simulink model "taghriban_kamel_faghat_bare3yekam_Ero"  (Simulink 7.3)
settings: Solver=ode45  StartTime=0.0  StopTime=.6  RelTol=1e-3
undefined symbols (not defined in the file or in its folder): x
libraries: powerlib x218, powerlib_extras x125
(part 1 of 2)
settings Model: Creator=me  LastModifiedBy=me

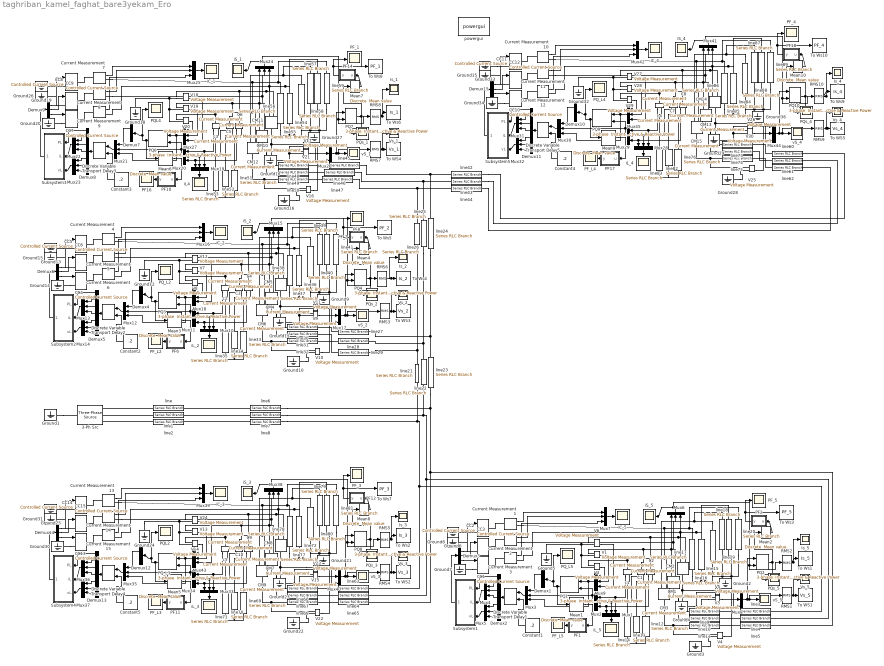
== system taghriban_kamel_faghat_bare3yekam_Ero ==
  3-Ph Src : powerlib/Electrical Sources/Three-Phase Source  DialogController=POWERSYS.PowerSysDialog  SystemSampleTime=-1  Voltage=380  PhaseAngle=0  Frequency=50  InternalConnection=Yn  SpecifyImpedance=on  Resistance=0.8929  Inductance=16.58e-3  ShortCircuitLevel=100e6  BaseVoltage=380  XRratio=7
  C{1..10} (10 alike) : powerlib/Measurements/Current Measurement  DialogController=POWERSYS.PowerSysDialog  SystemSampleTime=-1  PhasorSimulation=off  OutputType=Complex  PSBequivalent=0
  CC{1..15} (15 alike) : powerlib/Electrical Sources/Controlled Current Source  DialogController=POWERSYS.PowerSysDialog  SystemSampleTime=-1  Initialize=on  Source_Type=AC  Amplitude=0  Phase=0  Frequency=0  Measurements=None
  CM{1..15} (15 alike) : powerlib/Measurements/Current Measurement  DialogController=POWERSYS.PowerSysDialog  SystemSampleTime=-1  PhasorSimulation=off  OutputType=Complex  PSBequivalent=0
  Constant{1..5} (5 alike) : Constant  Value=.2  OutDataType=sfix(16)  OutScaling=2^0
  Current Measurement{1..15} (15 alike) : powerlib/Measurements/Current Measurement  DialogController=POWERSYS.PowerSysDialog  SystemSampleTime=-1  PhasorSimulation=off  OutputType=Complex  PSBequivalent=0
  Demux{1,4,7,10,12} (5 alike) : Demux  Outputs=2
  Demux{2,5,8,11,13} (5 alike) : Demux  Outputs=7
  Demux{3,6,9,14..15} (5 alike) : Demux  Outputs=3
  Discrete Variable Transport Delay{1..5} (5 alike) : powerlib_extras/Discrete  Control Blocks/Discrete Variable Transport Delay  DialogController=POWERSYS.PowerSysDialog  SystemSampleTime=-1  MaxDelay=1/40  InitialValue=0  Ts=50e-6
  Ground{1..36} (36 alike) : powerlib/Elements/Ground  DialogController=POWERSYS.PowerSysDialog  PhysicalDomain=powersysdomain  SubClassName=unknown  LeftPortType=p1  RightPortType=p1  LConnTagsString=a
  Is_{1..5} (5 alike) : Scope
      Is_1 settings: TimeRange=0.25  YMin=-1  YMax=1  SaveName=ScopeData21
      Is_2 settings: TimeRange=0.25  YMin=-1  YMax=1  SaveName=ScopeData11
      Is_3 settings: TimeRange=0.25  YMin=-1  YMax=1  SaveName=ScopeData50
      Is_4 settings: TimeRange=0.25  YMin=-1  YMax=1  SaveName=ScopeData44
      Is_5 settings: TimeRange=0.25  YMin=-1  YMax=1
  Mean{1..10} (10 alike) : powerlib_extras/Discrete Measurements/Discrete  Mean value  DialogController=POWERSYS.PowerSysDialog  SystemSampleTime=-1  Freq=60  Vinit=0  Ts=50e-6
  Mux{1..45} (45 alike) : Mux  Inputs=3
  PF1 : Stateflow chart
  PF10 : Stateflow chart
  PF11 : Stateflow chart
  PF12 : Stateflow chart
  PF14 : Stateflow chart
  PF16 : Scope
      settings: YMin=0.9675  YMax=0.9975  SaveName=ScopeData28
  PF17 : Stateflow chart
  PF18 : Stateflow chart
  PF2 : Stateflow chart
  PF6 : Stateflow chart
  PF8 : Scope
      settings: YMin=0.9961  YMax=0.9978  SaveName=ScopeData12
  PF_{1,3..5} (4 alike) : Scope
      PF_1 settings: YMin=0.957  YMax=0.965  SaveName=ScopeData22
      PF_3 settings: YMin=0.9961  YMax=0.9978  SaveName=ScopeData23
      PF_4 settings: YMin=0.9961  YMax=0.9978  SaveName=ScopeData45
      PF_5 settings: YMin=0.9961  YMax=0.9978  SaveName=ScopeData2
  PF_2 : Stateflow chart
  PF_L{2..5} (4 alike) : Scope
      PF_L2 settings: YMin=0.9675  YMax=0.9975  SaveName=ScopeData13
      PF_L3 settings: YMin=0.9675  YMax=0.9975  SaveName=ScopeData24
      PF_L4 settings: YMin=0.9675  YMax=0.9975  SaveName=ScopeData46
      PF_L5 settings: YMin=0.9675  YMax=0.9975  SaveName=ScopeData3
  PQ{1..4,6..10} (9 alike) : powerlib_extras/Measurements/3-phase  Instantaneous  Active & Reactive Power  DialogController=POWERSYS.PowerSysDialog  SystemSampleTime=-1
  PQL2 : Scope
      settings: TimeRange=0.2  YMin=-2e+008  YMax=9e+008  SaveName=ScopeData25
  PQL4 : Scope
      settings: TimeRange=0.2  YMin=-2e+008  YMax=9e+008  SaveName=ScopeData29
  PQ_L2 : Scope
      settings: TimeRange=0.2  YMin=-2e+008  YMax=9e+008  SaveName=ScopeData14
  PQ_L3 : powerlib_extras/Measurements/3-phase  Instantaneous  Active & Reactive Power  DialogController=POWERSYS.PowerSysDialog  SystemSampleTime=-1
  PQ_L4 : Scope
      settings: TimeRange=0.2  YMin=-2e+008  YMax=9e+008  SaveName=ScopeData47
  PQ_L5 : Scope
      settings: TimeRange=0.2  YMin=-2e+008  YMax=9e+008  SaveName=ScopeData4
  PQs_{1..5} (5 alike) : Scope
      PQs_1 settings: TimeRange=0.25  YMin=-250  YMax=4000  SaveName=ScopeData30
      PQs_2 settings: TimeRange=0.25  YMin=-250  YMax=4000  SaveName=ScopeData15
      PQs_3 settings: TimeRange=0.25  YMin=-250  YMax=4000  SaveName=ScopeData26
      PQs_4 settings: TimeRange=0.25  YMin=-250  YMax=4000  SaveName=ScopeData48
      PQs_5 settings: TimeRange=0.25  YMin=-250  YMax=4000  SaveName=ScopeData5
  RMS{1..10} (10 alike) : powerlib_extras/Measurements/RMS  DialogController=POWERSYS.PowerSysDialog  SystemSampleTime=-1  f1=50
  Subsystem1 : Subsystem
  Subsystem2 : Subsystem
  Subsystem3 : Subsystem
  Subsystem4 : Subsystem
  Subsystem5 : Subsystem
  To WS1 : ToWorkspace  VariableName=Vs_5  SampleTime=.01  SaveFormat=Array
  To WS2 : ToWorkspace  VariableName=Vs_3  SampleTime=.01  SaveFormat=Array
  To WS3 : ToWorkspace  VariableName=Vs_2  SampleTime=.01  SaveFormat=Array
  To WS4 : ToWorkspace  VariableName=Vs_1  SampleTime=.01  SaveFormat=Array
  To WS5 : ToWorkspace  VariableName=Vs_4  SampleTime=.01  SaveFormat=Array
  To Ws1 : ToWorkspace  VariableName=Is_5  SampleTime=.01  SaveFormat=Array
  To Ws10 : ToWorkspace  VariableName=PF_4  SampleTime=.01  SaveFormat=Array
  To Ws2 : ToWorkspace  VariableName=Is_3  SampleTime=.01  SaveFormat=Array
  To Ws3 : ToWorkspace  VariableName=PF_5  SampleTime=.01  SaveFormat=Array
  To Ws4 : ToWorkspace  VariableName=Is_2  SampleTime=.01  SaveFormat=Array
  To Ws5 : ToWorkspace  VariableName=PF_2  SampleTime=.01  SaveFormat=Array
  To Ws6 : ToWorkspace  VariableName=Is_1  SampleTime=.01  SaveFormat=Array
  To Ws7 : ToWorkspace  VariableName=PF_3  SampleTime=.01  SaveFormat=Array
  To Ws8 : ToWorkspace  VariableName=PF_1  SampleTime=.01  SaveFormat=Array
  To Ws9 : ToWorkspace  VariableName=Is_4  SampleTime=.01  SaveFormat=Array
  V{1..30} (30 alike) : powerlib/Measurements/Voltage Measurement  DialogController=POWERSYS.PowerSysDialog  SystemSampleTime=-1  PhasorSimulation=off  OutputType=Complex  PSBequivalent=0
  Vs_{1..5} (5 alike) : Scope
      Vs_1 settings: TimeRange=0.25  YMin=217.8  YMax=217.93  SaveName=ScopeData36
      Vs_2 settings: TimeRange=0.25  YMin=217.8  YMax=217.93  SaveName=ScopeData16
      Vs_3 settings: TimeRange=0.25  YMin=217.8  YMax=217.93  SaveName=ScopeData51
      Vs_4 settings: TimeRange=0.25  YMin=217.8  YMax=217.93  SaveName=ScopeData49
      Vs_5 settings: TimeRange=0.25  YMin=217.8  YMax=217.93  SaveName=ScopeData6
  c{1..5} (5 alike) : powerlib/Measurements/Current Measurement  DialogController=POWERSYS.PowerSysDialog  SystemSampleTime=-1  PhasorSimulation=off  OutputType=Complex  PSBequivalent=0
  iC_{1..5} (5 alike) : Scope
      iC_1 settings: TimeRange=0.15  YMin=-10  YMax=10  SaveName=ScopeData38
      iC_2 settings: TimeRange=0.15  YMin=-10  YMax=10  SaveName=ScopeData17
      iC_3 settings: TimeRange=0.15  YMin=-10  YMax=10  SaveName=ScopeData27
      iC_4 settings: TimeRange=0.15  YMin=-10  YMax=10  SaveName=ScopeData52
      iC_5 settings: TimeRange=0.15  YMin=-10  YMax=10  SaveName=ScopeData7
  iL4 : Scope
      settings: TimeRange=0.15  YMin=-4000  YMax=3500  SaveName=ScopeData39
  iL_{2..5} (4 alike) : Scope
      iL_2 settings: TimeRange=0.15  YMin=-4000  YMax=3500  SaveName=ScopeData18
      iL_3 settings: TimeRange=0.15  YMin=-4000  YMax=3500  SaveName=ScopeData37
      iL_4 settings: TimeRange=0.15  YMin=-4000  YMax=3500  SaveName=ScopeData53
      iL_5 settings: TimeRange=0.15  YMin=-4000  YMax=3500  SaveName=ScopeData8
  iS_{1..5} (5 alike) : Scope
      iS_1 settings: TimeRange=0.2  YMin=-15  YMax=15  SaveName=ScopeData42
      iS_2 settings: TimeRange=0.2  YMin=-17.5  YMax=17.5  SaveName=ScopeData19
      iS_3 settings: TimeRange=0.25  YMin=-15  YMax=15  SaveName=ScopeData40
      iS_4 settings: TimeRange=0.45  YMin=-10  YMax=10  SaveName=ScopeData54
      iS_5 settings: TimeRange=0.45  YMin=-12.5  YMax=12.5  SaveName=ScopeData9
  line : powerlib/Elements/Series RLC Branch  DialogController=POWERSYS.PowerSysDialog  PhysicalDomain=powersysdomain  SubClassName=unknown  LeftPortType=p1  RightPortType=p1  LConnTagsString=__new0  RConnTagsString=__new0  BranchType=RL  Resistance=.08  Inductance=.06/(100*pi)  SetiL0=off  InitialCurrent=0  Capacitance=1.0  Setx0=off  InitialVoltage=0  Measurements=None
  line1 : powerlib/Elements/Series RLC Branch  DialogController=POWERSYS.PowerSysDialog  PhysicalDomain=powersysdomain  SubClassName=unknown  LeftPortType=p1  RightPortType=p1  LConnTagsString=__new0  RConnTagsString=__new0  BranchType=RL  Resistance=.08  Inductance=.06/(100*pi)  SetiL0=off  InitialCurrent=0  Capacitance=1.0  Setx0=off  InitialVoltage=0  Measurements=None
  line{9..11,30..32,48..50,66..68,73..75} (15 alike) : powerlib/Elements/Series RLC Branch  DialogController=POWERSYS.PowerSysDialog  PhysicalDomain=powersysdomain  SubClassName=unknown  LeftPortType=p1  RightPortType=p1  LConnTagsString=__new0  RConnTagsString=__new0  BranchType=RL  Resistance=.1  Inductance=.08/(100*pi)  SetiL0=off  InitialCurrent=0  Capacitance=1.0  Setx0=off  InitialVoltage=0  Measurements=None
  line12 : powerlib/Elements/Series RLC Branch  DialogController=POWERSYS.PowerSysDialog  PhysicalDomain=powersysdomain  SubClassName=unknown  LeftPortType=p1  RightPortType=p1  LConnTagsString=__new0  RConnTagsString=__new0  BranchType=RL  Resistance=24  Inductance=19/(100*pi)  SetiL0=off  InitialCurrent=0  Capacitance=1.0  Setx0=off  InitialVoltage=0  Measurements=None
  line13 : powerlib/Elements/Series RLC Branch  DialogController=POWERSYS.PowerSysDialog  PhysicalDomain=powersysdomain  SubClassName=unknown  LeftPortType=p1  RightPortType=p1  LConnTagsString=__new0  RConnTagsString=__new0  BranchType=Open circuit  Resistance=50  Inductance=50/(100*pi)  SetiL0=off  InitialCurrent=0  Capacitance=1/(100*pi)  Setx0=off  InitialVoltage=0  Measurements=None
  line14 : powerlib/Elements/Series RLC Branch  DialogController=POWERSYS.PowerSysDialog  PhysicalDomain=powersysdomain  SubClassName=unknown  LeftPortType=p1  RightPortType=p1  LConnTagsString=__new0  RConnTagsString=__new0  BranchType=RL  Resistance=10  Inductance=30/(100*pi)  SetiL0=off  InitialCurrent=0  Capacitance=1/(100*pi)  Setx0=off  InitialVoltage=0  Measurements=None
  line{15..17,36..38,54..56,72,77..78,84..86} (15 alike) : powerlib/Elements/Series RLC Branch  DialogController=POWERSYS.PowerSysDialog  PhysicalDomain=powersysdomain  SubClassName=unknown  LeftPortType=p1  RightPortType=p1  LConnTagsString=__new0  RConnTagsString=__new0  BranchType=R  Resistance=100  Inductance=.04/(100*pi)  SetiL0=off  InitialCurrent=0  Capacitance=1.0  Setx0=off  InitialVoltage=0  Measurements=None
  line{18..20,39..41,57..59,79..81,87..89} (15 alike) : powerlib/Elements/Series RLC Branch  DialogController=POWERSYS.PowerSysDialog  PhysicalDomain=powersysdomain  SubClassName=unknown  LeftPortType=p1  RightPortType=p1  LConnTagsString=__new0  RConnTagsString=__new0  BranchType=C  Resistance=100  Inductance=.04/(100*pi)  SetiL0=off  InitialCurrent=0  Capacitance=1/(10000*pi)  Setx0=off  InitialVoltage=0  Measurements=None
  line2 : powerlib/Elements/Series RLC Branch  DialogController=POWERSYS.PowerSysDialog  PhysicalDomain=powersysdomain  SubClassName=unknown  LeftPortType=p1  RightPortType=p1  LConnTagsString=__new0  RConnTagsString=__new0  BranchType=RL  Resistance=.08  Inductance=.06/(100*pi)  SetiL0=off  InitialCurrent=0  Capacitance=1.0  Setx0=off  InitialVoltage=0  Measurements=None
  line21 : powerlib/Elements/Series RLC Branch  DialogController=POWERSYS.PowerSysDialog  PhysicalDomain=powersysdomain  SubClassName=unknown  LeftPortType=p1  RightPortType=p1  LConnTagsString=__new0  RConnTagsString=__new0  BranchType=RL  Resistance=.11  Inductance=.08/(100*pi)  SetiL0=off  InitialCurrent=0  Capacitance=1.0  Setx0=off  InitialVoltage=0  Measurements=None
  line22 : powerlib/Elements/Series RLC Branch  DialogController=POWERSYS.PowerSysDialog  PhysicalDomain=powersysdomain  SubClassName=unknown  LeftPortType=p1  RightPortType=p1  LConnTagsString=__new0  RConnTagsString=__new0  BranchType=RL  Resistance=.11  Inductance=.08/(100*pi)  SetiL0=off  InitialCurrent=0  Capacitance=1.0  Setx0=off  InitialVoltage=0  Measurements=None
  line23 : powerlib/Elements/Series RLC Branch  DialogController=POWERSYS.PowerSysDialog  PhysicalDomain=powersysdomain  SubClassName=unknown  LeftPortType=p1  RightPortType=p1  LConnTagsString=__new0  RConnTagsString=__new0  BranchType=RL  Resistance=.11  Inductance=.08/(100*pi)  SetiL0=off  InitialCurrent=0  Capacitance=1.0  Setx0=off  InitialVoltage=0  Measurements=None
  line24 : powerlib/Elements/Series RLC Branch  DialogController=POWERSYS.PowerSysDialog  PhysicalDomain=powersysdomain  SubClassName=unknown  LeftPortType=p1  RightPortType=p1  LConnTagsString=__new0  RConnTagsString=__new0  BranchType=RL  Resistance=.06  Inductance=.04/(100*pi)  SetiL0=off  InitialCurrent=0  Capacitance=1.0  Setx0=off  InitialVoltage=0  Measurements=None
  line25 : powerlib/Elements/Series RLC Branch  DialogController=POWERSYS.PowerSysDialog  PhysicalDomain=powersysdomain  SubClassName=unknown  LeftPortType=p1  RightPortType=p1  LConnTagsString=__new0  RConnTagsString=__new0  BranchType=RL  Resistance=.06  Inductance=.04/(100*pi)  SetiL0=off  InitialCurrent=0  Capacitance=1.0  Setx0=off  InitialVoltage=0  Measurements=None
  line26 : powerlib/Elements/Series RLC Branch  DialogController=POWERSYS.PowerSysDialog  PhysicalDomain=powersysdomain  SubClassName=unknown  LeftPortType=p1  RightPortType=p1  LConnTagsString=__new0  RConnTagsString=__new0  BranchType=RL  Resistance=.06  Inductance=.04/(100*pi)  SetiL0=off  InitialCurrent=0  Capacitance=1.0  Setx0=off  InitialVoltage=0  Measurements=None
  line{3,27,45,60,63} (5 alike) : powerlib/Elements/Series RLC Branch  DialogController=POWERSYS.PowerSysDialog  PhysicalDomain=powersysdomain  SubClassName=unknown  LeftPortType=p1  RightPortType=p1  LConnTagsString=__new0  RConnTagsString=__new0  BranchType=R  Resistance=.000000000001  Inductance=1.0  SetiL0=off  InitialCurrent=0  Capacitance=1.0  Setx0=off  InitialVoltage=0  Measurements=None
  line{4,28,46,61,64} (5 alike) : powerlib/Elements/Series RLC Branch  DialogController=POWERSYS.PowerSysDialog  PhysicalDomain=powersysdomain  SubClassName=unknown  LeftPortType=p1  RightPortType=p1  LConnTagsString=__new0  RConnTagsString=__new0  BranchType=R  Resistance=.0000000001  Inductance=1.0  SetiL0=off  InitialCurrent=0  Capacitance=1.0  Setx0=off  InitialVoltage=0  Measurements=None
  line{5,29,47,62,65} (5 alike) : powerlib/Elements/Series RLC Branch  DialogController=POWERSYS.PowerSysDialog  PhysicalDomain=powersysdomain  SubClassName=unknown  LeftPortType=p1  RightPortType=p1  LConnTagsString=__new0  RConnTagsString=__new0  BranchType=R  Resistance=.0000000000001  Inductance=1.0  SetiL0=off  InitialCurrent=0  Capacitance=1.0  Setx0=off  InitialVoltage=0  Measurements=None
  line33 : powerlib/Elements/Series RLC Branch  DialogController=POWERSYS.PowerSysDialog  PhysicalDomain=powersysdomain  SubClassName=unknown  LeftPortType=p1  RightPortType=p1  LConnTagsString=__new0  RConnTagsString=__new0  BranchType=RL  Resistance=14  Inductance=29/(100*pi)  SetiL0=off  InitialCurrent=0  Capacitance=1.0  Setx0=off  InitialVoltage=0  Measurements=None
  line34 : powerlib/Elements/Series RLC Branch  DialogController=POWERSYS.PowerSysDialog  PhysicalDomain=powersysdomain  SubClassName=unknown  LeftPortType=p1  RightPortType=p1  LConnTagsString=__new0  RConnTagsString=__new0  BranchType=RC  Resistance=23  Inductance=50/(100*pi)  SetiL0=off  InitialCurrent=0  Capacitance=1/(1200*pi)  Setx0=off  InitialVoltage=0  Measurements=None
  line35 : powerlib/Elements/Series RLC Branch  DialogController=POWERSYS.PowerSysDialog  PhysicalDomain=powersysdomain  SubClassName=unknown  LeftPortType=p1  RightPortType=p1  LConnTagsString=__new0  RConnTagsString=__new0  BranchType=Open circuit  Resistance=10  Inductance=30/(100*pi)  SetiL0=off  InitialCurrent=0  Capacitance=1/(100*pi)  Setx0=off  InitialVoltage=0  Measurements=None
  line42 : powerlib/Elements/Series RLC Branch  DialogController=POWERSYS.PowerSysDialog  PhysicalDomain=powersysdomain  SubClassName=unknown  LeftPortType=p1  RightPortType=p1  LConnTagsString=__new0  RConnTagsString=__new0  BranchType=RL  Resistance=.05  Inductance=.04/(100*pi)  SetiL0=off  InitialCurrent=0  Capacitance=1.0  Setx0=off  InitialVoltage=0  Measurements=None
  line43 : powerlib/Elements/Series RLC Branch  DialogController=POWERSYS.PowerSysDialog  PhysicalDomain=powersysdomain  SubClassName=unknown  LeftPortType=p1  RightPortType=p1  LConnTagsString=__new0  RConnTagsString=__new0  BranchType=RL  Resistance=.05  Inductance=.04/(100*pi)  SetiL0=off  InitialCurrent=0  Capacitance=1.0  Setx0=off  InitialVoltage=0  Measurements=None
  line44 : powerlib/Elements/Series RLC Branch  DialogController=POWERSYS.PowerSysDialog  PhysicalDomain=powersysdomain  SubClassName=unknown  LeftPortType=p1  RightPortType=p1  LConnTagsString=__new0  RConnTagsString=__new0  BranchType=RL  Resistance=.05  Inductance=.04/(100*pi)  SetiL0=off  InitialCurrent=0  Capacitance=1.0  Setx0=off  InitialVoltage=0  Measurements=None
  line51 : powerlib/Elements/Series RLC Branch  DialogController=POWERSYS.PowerSysDialog  PhysicalDomain=powersysdomain  SubClassName=unknown  LeftPortType=p1  RightPortType=p1  LConnTagsString=__new0  RConnTagsString=__new0  BranchType=RLC  Resistance=24  Inductance=39/(100*pi)  SetiL0=off  InitialCurrent=0  Capacitance=1/(1200*pi)  Setx0=off  InitialVoltage=0  Measurements=None
  line52 : powerlib/Elements/Series RLC Branch  DialogController=POWERSYS.PowerSysDialog  PhysicalDomain=powersysdomain  SubClassName=unknown  LeftPortType=p1  RightPortType=p1  LConnTagsString=__new0  RConnTagsString=__new0  BranchType=RC  Resistance=50  Inductance=50/(100*pi)  SetiL0=off  InitialCurrent=0  Capacitance=1/(1000*pi)  Setx0=off  InitialVoltage=0  Measurements=None
  line53 : powerlib/Elements/Series RLC Branch  DialogController=POWERSYS.PowerSysDialog  PhysicalDomain=powersysdomain  SubClassName=unknown  LeftPortType=p1  RightPortType=p1  LConnTagsString=__new0  RConnTagsString=__new0  BranchType=RL  Resistance=5  Inductance=30/(100*pi)  SetiL0=off  InitialCurrent=0  Capacitance=1/(100*pi)  Setx0=off  InitialVoltage=0  Measurements=None
  line6 : powerlib/Elements/Series RLC Branch  DialogController=POWERSYS.PowerSysDialog  PhysicalDomain=powersysdomain  SubClassName=unknown  LeftPortType=p1  RightPortType=p1  LConnTagsString=__new0  RConnTagsString=__new0  BranchType=RL  Resistance=.03  Inductance=.02/(100*pi)  SetiL0=off  InitialCurrent=0  Capacitance=1.0  Setx0=off  InitialVoltage=0  Measurements=None
  line69 : powerlib/Elements/Series RLC Branch  DialogController=POWERSYS.PowerSysDialog  PhysicalDomain=powersysdomain  SubClassName=unknown  LeftPortType=p1  RightPortType=p1  LConnTagsString=__new0  RConnTagsString=__new0  BranchType=RL  Resistance=24  Inductance=9/(100*pi)  SetiL0=off  InitialCurrent=0  Capacitance=1.0  Setx0=off  InitialVoltage=0  Measurements=None
  line7 : powerlib/Elements/Series RLC Branch  DialogController=POWERSYS.PowerSysDialog  PhysicalDomain=powersysdomain  SubClassName=unknown  LeftPortType=p1  RightPortType=p1  LConnTagsString=__new0  RConnTagsString=__new0  BranchType=RL  Resistance=.03  Inductance=.02/(100*pi)  SetiL0=off  InitialCurrent=0  Capacitance=1.0  Setx0=off  InitialVoltage=0  Measurements=None
  line70 : powerlib/Elements/Series RLC Branch  DialogController=POWERSYS.PowerSysDialog  PhysicalDomain=powersysdomain  SubClassName=unknown  LeftPortType=p1  RightPortType=p1  LConnTagsString=__new0  RConnTagsString=__new0  BranchType=RLC  Resistance=15  Inductance=50/(100*pi)  SetiL0=off  InitialCurrent=0  Capacitance=26/(100*pi)  Setx0=off  InitialVoltage=0  Measurements=None
  line71 : powerlib/Elements/Series RLC Branch  DialogController=POWERSYS.PowerSysDialog  PhysicalDomain=powersysdomain  SubClassName=unknown  LeftPortType=p1  RightPortType=p1  LConnTagsString=__new0  RConnTagsString=__new0  BranchType=L  Resistance=10  Inductance=30/(100*pi)  SetiL0=off  InitialCurrent=0  Capacitance=1/(100*pi)  Setx0=off  InitialVoltage=0  Measurements=None
  line76 : powerlib/Elements/Series RLC Branch  DialogController=POWERSYS.PowerSysDialog  PhysicalDomain=powersysdomain  SubClassName=unknown  LeftPortType=p1  RightPortType=p1  LConnTagsString=__new0  RConnTagsString=__new0  BranchType=RL  Resistance=24  Inductance=41/(100*pi)  SetiL0=off  InitialCurrent=0  Capacitance=1.0  Setx0=off  InitialVoltage=0  Measurements=None
  line8 : powerlib/Elements/Series RLC Branch  DialogController=POWERSYS.PowerSysDialog  PhysicalDomain=powersysdomain  SubClassName=unknown  LeftPortType=p1  RightPortType=p1  LConnTagsString=__new0  RConnTagsString=__new0  BranchType=RL  Resistance=.03  Inductance=.02/(100*pi)  SetiL0=off  InitialCurrent=0  Capacitance=1.0  Setx0=off  InitialVoltage=0  Measurements=None
  line82 : powerlib/Elements/Series RLC Branch  DialogController=POWERSYS.PowerSysDialog  PhysicalDomain=powersysdomain  SubClassName=unknown  LeftPortType=p1  RightPortType=p1  LConnTagsString=__new0  RConnTagsString=__new0  BranchType=RLC  Resistance=7  Inductance=50/(100*pi)  SetiL0=off  InitialCurrent=0  Capacitance=1/(1000*pi)  Setx0=off  InitialVoltage=0  Measurements=None
  line83 : powerlib/Elements/Series RLC Branch  DialogController=POWERSYS.PowerSysDialog  PhysicalDomain=powersysdomain  SubClassName=unknown  LeftPortType=p1  RightPortType=p1  LConnTagsString=__new0  RConnTagsString=__new0  BranchType=RL  Resistance=10  Inductance=20/(100*pi)  SetiL0=off  InitialCurrent=0  Capacitance=1/(100*pi)  Setx0=off  InitialVoltage=0  Measurements=None
  powergui : powerlib/powergui  Priority=1  SystemSampleTime=-1  SimulationMode=Continuous  SampleTime=50e-6  frequency=60  SPID=off  DisableSnubberDevices=off  DisableRonSwitches=off  DisableVfSwitches=off  SwTol=0  Interpol=off  frequencyindice=50  echomessages=off  HookPort=off  DisplayEquations=off  FunctionMessages=off  EnableUseOfTLC=off  x0status=blocks  RestoreLinks=warning  Frange=[0:2:500]  Ylog=off  Xlog=on  ShowGrid=off  save=off  variable=ZData  ZoomFFT=on  StartTime=0.0  cycles=1  DisplayStyle=1  fundamental=60  FreqAxis=off  MaxFrequency=1000  frequencyindicesteady=1  RmsSteady=1  display=off  Ts=0  methode=off
  vS_{1..5} (5 alike) : Scope
      vS_1 settings: TimeRange=0.15  YMin=-350  YMax=250  SaveName=ScopeData43
      vS_2 settings: TimeRange=0.15  YMin=-350  YMax=250  SaveName=ScopeData20
      vS_3 settings: TimeRange=0.15  YMin=-350  YMax=250  SaveName=ScopeData41
      vS_4 settings: TimeRange=0.15  YMin=-350  YMax=250  SaveName=ScopeData55
      vS_5 settings: TimeRange=0.15  YMin=-350  YMax=250  SaveName=ScopeData10
  wires:
  V14/1 -> Mux43/1
  V13/1 -> Mux43/2
  V24/1 -> Mux43/3
  c5/1 -> Mux34/1, Mux33/3
  C10/1 -> Mux34/2, Mux33/2
  C9/1 -> Mux34/3, Mux33/1
  Mux34/1 -> PQ_L3/2, Mux35/2
  Mux43/1 -> Mux35/3, PQ_L3/1
  Mux33/1 -> iL_3/1
  Mean5/1 -> PF11/1(u)
  PF11/1(y) -> PF_L3/1
  PQ_L3/1 -> Mean5/1, PQL2/1, Demux12/1
  Demux12/1 -> Mux35/1
  Mux35/1 -> Discrete Variable Transport Delay4/1
  Discrete Variable Transport Delay4/1 -> Demux13/1
  Constant5/1 -> Discrete Variable Transport Delay4/2
  Demux13/5 -> Mux37/1
  Demux13/7 -> Mux37/3
  Demux13/6 -> Mux37/2
  Demux13/3 -> Mux36/2
  Demux13/2 -> Mux36/1
  Demux13/4 -> Mux36/3
  Demux14/1 -> CC14/1
  Demux14/2 -> CC15/1
  Demux14/3 -> CC13/1
  Subsystem4/1(Out1) -> Demux14/1
  CM9/1 -> Mux38/1
  CM7/1 -> Mux38/2
  CM8/1 -> Mux38/3
  Mux38/1 -> iS_3/1, PQ8/2, RMS5/1
  Mux39/1 -> iC_3/1
  Current Measurement13/1 -> Mux39/1
  Current Measurement14/1 -> Mux39/2
  Current Measurement15/1 -> Mux39/3
  Demux13/1 -> Subsystem4/1(PL)
  Mux36/1 -> Subsystem4/2(iL)
  Mux37/1 -> Subsystem4/3(vL)
  V22/1 -> Mux40/1
  V23/1 -> Mux40/2
  V15/1 -> Mux40/3
  Mux40/1 -> PQ8/1, vS_3/1, RMS4/1
  PQ8/1 -> PQs_3/1, Mean8/1
  PF12/1(y) -> PF_3/1, To Ws7/1
  Mean8/1 -> PF12/1(u)
  RMS4/1 -> Vs_3/1, To WS2/1
  RMS5/1 -> Is_3/1, To Ws2/1
  V2/1 -> Mux9/1
  V1/1 -> Mux9/2
  V6/1 -> Mux9/3
  c1/1 -> Mux2/1, Mux1/3
  C1/1 -> Mux2/2, Mux1/2
  C2/1 -> Mux2/3, Mux1/1
  Mux2/1 -> PQ1/2, Mux3/2
  Mux9/1 -> Mux3/3, PQ1/1
  Mux1/1 -> iL_5/1
  Mean1/1 -> PF1/1(u)
  PF1/1(y) -> PF_L5/1
  PQ1/1 -> Mean1/1, PQ_L5/1, Demux1/1
  Demux1/1 -> Mux3/1
  Mux3/1 -> Discrete Variable Transport Delay1/1
  Discrete Variable Transport Delay1/1 -> Demux2/1
  Constant1/1 -> Discrete Variable Transport Delay1/2
  Demux2/5 -> Mux5/1
  Demux2/7 -> Mux5/3
  Demux2/6 -> Mux5/2
  Demux2/3 -> Mux4/2
  Demux2/2 -> Mux4/1
  Demux2/4 -> Mux4/3
  Demux3/1 -> CC2/1
  Demux3/2 -> CC3/1
  Demux3/3 -> CC1/1
  Subsystem1/1(Out1) -> Demux3/1
  CM3/1 -> Mux6/1
  CM1/1 -> Mux6/2
  CM2/1 -> Mux6/3
  Mux6/1 -> iS_5/1, PQ2/2, RMS2/1
  Mux7/1 -> iC_5/1
  Current Measurement1/1 -> Mux7/1
  Current Measurement2/1 -> Mux7/2
  Current Measurement3/1 -> Mux7/3
  Demux2/1 -> Subsystem1/1(PL)
  Mux4/1 -> Subsystem1/2(iL)
  Mux5/1 -> Subsystem1/3(vL)
  V4/1 -> Mux8/1
  V5/1 -> Mux8/2
  V3/1 -> Mux8/3
  Mux8/1 -> PQ2/1, vS_5/1, RMS1/1
  PQ2/1 -> PQs_5/1, Mean2/1
  PF2/1(y) -> PF_5/1, To Ws3/1
  Mean2/1 -> PF2/1(u)
  RMS1/1 -> Vs_5/1, To WS1/1
  RMS2/1 -> Is_5/1, To Ws1/1
  V8/1 -> Mux18/1
  V7/1 -> Mux18/2
  V12/1 -> Mux18/3
  c2/1 -> Mux11/1, Mux10/3
  C3/1 -> Mux11/2, Mux10/2
  C4/1 -> Mux11/3, Mux10/1
  Mux11/1 -> PQ3/2, Mux12/2
  Mux18/1 -> Mux12/3, PQ3/1
  Mux10/1 -> iL_2/1
  Mean3/1 -> PF6/1(u)
  PF6/1(y) -> PF_L2/1
  PQ3/1 -> Mean3/1, PQ_L2/1, Demux4/1
  Demux4/1 -> Mux12/1
  Mux12/1 -> Discrete Variable Transport Delay2/1
  Discrete Variable Transport Delay2/1 -> Demux5/1
  Constant2/1 -> Discrete Variable Transport Delay2/2
  Demux5/5 -> Mux14/1
  Demux5/7 -> Mux14/3
  Demux5/6 -> Mux14/2
  Demux5/3 -> Mux13/2
  Demux5/2 -> Mux13/1
  Demux5/4 -> Mux13/3
  Demux6/1 -> CC5/1
  Demux6/2 -> CC6/1
  Demux6/3 -> CC4/1
  Subsystem2/1(Out1) -> Demux6/1
  CM6/1 -> Mux15/1
  CM4/1 -> Mux15/2
  CM5/1 -> Mux15/3
  Mux15/1 -> iS_2/1, PQ4/2, RMS6/1
  Mux16/1 -> iC_2/1
  Current Measurement4/1 -> Mux16/1
  Current Measurement5/1 -> Mux16/2
  Current Measurement6/1 -> Mux16/3
  Demux5/1 -> Subsystem2/1(PL)
  Mux13/1 -> Subsystem2/2(iL)
  Mux14/1 -> Subsystem2/3(vL)
  V10/1 -> Mux17/1
  V11/1 -> Mux17/2
  V9/1 -> Mux17/3
  Mux17/1 -> PQ4/1, vS_2/1, RMS3/1
  PQ4/1 -> PQs_2/1, Mean4/1
  PF_2/1(y) -> PF8/1, To Ws5/1
  Mean4/1 -> PF_2/1(u)
  RMS3/1 -> Vs_2/1, To WS3/1
  RMS6/1 -> Is_2/1, To Ws4/1
  V20/1 -> Mux27/1
  V19/1 -> Mux27/2
  V18/1 -> Mux27/3
  c3/1 -> Mux20/1, Mux19/3
  C5/1 -> Mux20/2, Mux19/2
  C6/1 -> Mux20/3, Mux19/1
  Mux20/1 -> PQ6/2, Mux21/2
  Mux27/1 -> Mux21/3, PQ6/1
  Mux19/1 -> iL4/1
  Mean6/1 -> PF10/1(u)
  PF10/1(y) -> PF16/1
  PQ6/1 -> Mean6/1, PQL4/1, Demux7/1
  Demux7/1 -> Mux21/1
  Mux21/1 -> Discrete Variable Transport Delay3/1
  Discrete Variable Transport Delay3/1 -> Demux8/1
  Constant3/1 -> Discrete Variable Transport Delay3/2
  Demux8/5 -> Mux23/1
  Demux8/7 -> Mux23/3
  Demux8/6 -> Mux23/2
  Demux8/3 -> Mux22/2
  Demux8/2 -> Mux22/1
  Demux8/4 -> Mux22/3
  Demux9/1 -> CC8/1
  Demux9/2 -> CC9/1
  Demux9/3 -> CC7/1
  Subsystem3/1(Out1) -> Demux9/1
  CM12/1 -> Mux24/1
  CM10/1 -> Mux24/2
  CM11/1 -> Mux24/3
  Mux24/1 -> iS_1/1, PQ7/2, RMS8/1
  Mux25/1 -> iC_1/1
  Current Measurement7/1 -> Mux25/1
  Current Measurement8/1 -> Mux25/2
  Current Measurement9/1 -> Mux25/3
  Demux8/1 -> Subsystem3/1(PL)
  Mux22/1 -> Subsystem3/2(iL)
  Mux23/1 -> Subsystem3/3(vL)
  V16/1 -> Mux26/1
  V17/1 -> Mux26/2
  V21/1 -> Mux26/3
  Mux26/1 -> PQ7/1, vS_1/1, RMS7/1
  PQ7/1 -> PQs_1/1, Mean7/1
  PF14/1(y) -> PF_1/1, To Ws8/1
  Mean7/1 -> PF14/1(u)
  RMS7/1 -> Vs_1/1, To WS4/1
  RMS8/1 -> Is_1/1, To Ws6/1
  V29/1 -> Mux45/1
  V28/1 -> Mux45/2
  V27/1 -> Mux45/3
  c4/1 -> Mux29/1, Mux28/3
  C7/1 -> Mux29/2, Mux28/2
  C8/1 -> Mux29/3, Mux28/1
  Mux29/1 -> PQ9/2, Mux30/2
  Mux45/1 -> Mux30/3, PQ9/1
  Mux28/1 -> iL_4/1
  Mean9/1 -> PF17/1(u)
  PF17/1(y) -> PF_L4/1
  PQ9/1 -> Mean9/1, PQ_L4/1, Demux10/1
  Demux10/1 -> Mux30/1
  Mux30/1 -> Discrete Variable Transport Delay5/1
  Discrete Variable Transport Delay5/1 -> Demux11/1
  Constant4/1 -> Discrete Variable Transport Delay5/2
  Demux11/5 -> Mux32/1
  Demux11/7 -> Mux32/3
  Demux11/6 -> Mux32/2
  Demux11/3 -> Mux31/2
  Demux11/2 -> Mux31/1
  Demux11/4 -> Mux31/3
  Demux15/1 -> CC11/1
  Demux15/2 -> CC12/1
  Demux15/3 -> CC10/1
  Subsystem5/1(Out1) -> Demux15/1
  CM15/1 -> Mux41/1
  CM13/1 -> Mux41/2
  CM14/1 -> Mux41/3
  Mux41/1 -> iS_4/1, PQ10/2, RMS10/1
  Mux42/1 -> iC_4/1
  Current Measurement10/1 -> Mux42/1
  Current Measurement11/1 -> Mux42/2
  Current Measurement12/1 -> Mux42/3
  Demux11/1 -> Subsystem5/1(PL)
  Mux31/1 -> Subsystem5/2(iL)
  Mux32/1 -> Subsystem5/3(vL)
  V25/1 -> Mux44/1
  V26/1 -> Mux44/2
  V30/1 -> Mux44/3
  Mux44/1 -> PQ10/1, vS_4/1, RMS9/1
  PQ10/1 -> PQs_4/1, Mean10/1
  PF18/1(y) -> PF_4/1, To Ws10/1
  Mean10/1 -> PF18/1(u)
  RMS9/1 -> Vs_4/1, To WS5/1
  RMS10/1 -> Is_4/1, To Ws9/1
  connections:
  line/LConn1 -- 3-Ph Src/RConn1
  line1/LConn1 -- 3-Ph Src/RConn2
  line2/LConn1 -- 3-Ph Src/RConn3
  line6/LConn1 -- line/RConn1
  line7/LConn1 -- line1/RConn1
  line8/LConn1 -- line2/RConn1
  line6/RConn1 -- line65/RConn1 -- line5/RConn1 -- line23/RConn1
  line7/RConn1 -- line64/RConn1 -- line4/RConn1 -- line22/RConn1
  line8/RConn1 -- line63/RConn1 -- line3/RConn1 -- line21/RConn1
  Ground24/LConn1 -- V24/LConn2 -- V14/LConn2 -- V13/LConn2
  line70/RConn1 -- line71/RConn1 -- line69/RConn1
  line80/LConn1 -- Current Measurement15/RConn1 -- V24/LConn1 -- C9/LConn1 -- CM8/RConn1 -- line77/LConn1
  line81/LConn1 -- V14/LConn1 -- c5/LConn1 -- CM9/RConn1 -- Current Measurement13/RConn1 -- line78/LConn1
  V13/LConn1 -- C10/LConn1 -- CM7/RConn1 -- Current Measurement14/RConn1 -- line79/LConn1 -- line72/LConn1
  line81/RConn1 -- line72/RConn1 -- Ground21/LConn1 -- line78/RConn1 -- line77/RConn1 -- line79/RConn1 -- line80/RConn1
  V23/LConn1 -- CM7/LConn1 -- line67/RConn1
  V15/LConn1 -- CM8/LConn1 -- line66/RConn1
  V22/LConn1 -- CM9/LConn1 -- line68/RConn1
  V15/LConn2 -- Ground23/LConn1 -- V23/LConn2
  line64/LConn1 -- line67/LConn1
  C9/RConn1 -- line69/LConn1
  line65/LConn1 -- line68/LConn1
  Current Measurement15/LConn1 -- CC13/RConn1
  Current Measurement14/LConn1 -- CC15/RConn1
  C10/RConn1 -- line70/LConn1
  Ground30/LConn1 -- CC13/LConn1
  Ground25/LConn1 -- CC14/LConn1
  CC15/LConn1 -- Ground31/LConn1
  Ground22/LConn1 -- V22/LConn2
  c5/RConn1 -- line71/LConn1
  line63/LConn1 -- line66/LConn1
  Current Measurement13/LConn1 -- CC14/RConn1
  Ground1/LConn1 -- 3-Ph Src/LConn1
  V1/LConn2 -- V2/LConn2 -- Ground5/LConn1 -- V6/LConn2
  line12/RConn1 -- line13/RConn1 -- line14/RConn1
  line16/LConn1 -- line19/LConn1 -- Current Measurement3/RConn1 -- V6/LConn1 -- C2/LConn1 -- CM2/RConn1
  line17/LConn1 -- line20/LConn1 -- V2/LConn1 -- c1/LConn1 -- CM3/RConn1 -- Current Measurement1/RConn1
  line15/LConn1 -- line18/LConn1 -- Current Measurement2/RConn1 -- CM1/RConn1 -- V1/LConn1 -- C1/LConn1
  line19/RConn1 -- line20/RConn1 -- line15/RConn1 -- Ground2/LConn1 -- line17/RConn1 -- line16/RConn1 -- line18/RConn1
  line10/RConn1 -- V5/LConn1 -- CM1/LConn1
  line9/RConn1 -- V3/LConn1 -- CM2/LConn1
  line11/RConn1 -- V4/LConn1 -- CM3/LConn1
  V5/LConn2 -- V3/LConn2 -- Ground4/LConn1
  line4/LConn1 -- line10/LConn1
  C2/RConn1 -- line12/LConn1
  line5/LConn1 -- line11/LConn1
  Current Measurement3/LConn1 -- CC1/RConn1
  Current Measurement2/LConn1 -- CC3/RConn1
  C1/RConn1 -- line13/LConn1
  Ground7/LConn1 -- CC1/LConn1
  Ground6/LConn1 -- CC2/LConn1
  CC3/LConn1 -- Ground8/LConn1
  Ground3/LConn1 -- V4/LConn2
  c1/RConn1 -- line14/LConn1
  line3/LConn1 -- line9/LConn1
  Current Measurement1/LConn1 -- CC2/RConn1
  line29/RConn1 -- line21/LConn1 -- line26/RConn1
  line28/RConn1 -- line22/LConn1 -- line25/RConn1
  line27/RConn1 -- line23/LConn1 -- line24/RConn1
  V7/LConn2 -- V8/LConn2 -- Ground12/LConn1 -- V12/LConn2
  line33/RConn1 -- line34/RConn1 -- line35/RConn1
  line37/LConn1 -- line40/LConn1 -- Current Measurement6/RConn1 -- V12/LConn1 -- C4/LConn1 -- CM5/RConn1
  line38/LConn1 -- line41/LConn1 -- V8/LConn1 -- c2/LConn1 -- CM6/RConn1 -- Current Measurement4/RConn1
  line36/LConn1 -- line39/LConn1 -- Current Measurement5/RConn1 -- CM4/RConn1 -- V7/LConn1 -- C3/LConn1
  line40/RConn1 -- line41/RConn1 -- line36/RConn1 -- Ground9/LConn1 -- line38/RConn1 -- line37/RConn1 -- line39/RConn1
  line31/RConn1 -- V11/LConn1 -- CM4/LConn1
  line30/RConn1 -- V9/LConn1 -- CM5/LConn1
  line32/RConn1 -- V10/LConn1 -- CM6/LConn1
  V11/LConn2 -- Ground11/LConn1 -- V9/LConn2
  line28/LConn1 -- line31/LConn1
  C4/RConn1 -- line33/LConn1
  line29/LConn1 -- line32/LConn1
  Current Measurement6/LConn1 -- CC4/RConn1
  Current Measurement5/LConn1 -- CC6/RConn1
  C3/RConn1 -- line34/LConn1
  Ground14/LConn1 -- CC4/LConn1
  Ground13/LConn1 -- CC5/LConn1
  CC6/LConn1 -- Ground15/LConn1
  Ground10/LConn1 -- V10/LConn2
  c2/RConn1 -- line35/LConn1
  line27/LConn1 -- line30/LConn1
  Current Measurement4/LConn1 -- CC5/RConn1
  line42/RConn1 -- line60/RConn1
  line44/RConn1 -- line62/RConn1
  line43/RConn1 -- line61/RConn1
  V18/LConn2 -- Ground18/LConn1 -- V20/LConn2 -- V19/LConn2
  line51/RConn1 -- line52/RConn1 -- line53/RConn1
  line55/LConn1 -- line58/LConn1 -- Current Measurement9/RConn1 -- CM11/RConn1 -- V18/LConn1 -- C6/LConn1
  line56/LConn1 -- line59/LConn1 -- Current Measurement7/RConn1 -- CM12/RConn1 -- V20/LConn1 -- c3/LConn1
  C5/LConn1 -- V19/LConn1 -- CM10/RConn1 -- Current Measurement8/RConn1 -- line57/LConn1 -- line54/LConn1
  line58/RConn1 -- line59/RConn1 -- line57/RConn1 -- line54/RConn1 -- Ground27/LConn1 -- line56/RConn1 -- line55/RConn1
  line49/RConn1 -- V17/LConn1 -- CM10/LConn1
  line48/RConn1 -- V21/LConn1 -- CM11/LConn1
  line50/RConn1 -- CM12/LConn1 -- V16/LConn1
  V17/LConn2 -- Ground17/LConn1 -- V21/LConn2
  CC9/LConn1 -- Ground26/LConn1
  Ground16/LConn1 -- V16/LConn2
  C5/RConn1 -- line52/LConn1
  Current Measurement8/LConn1 -- CC9/RConn1
  c3/RConn1 -- line53/LConn1
  line45/LConn1 -- line48/LConn1
  Ground20/LConn1 -- CC7/LConn1
  line46/LConn1 -- line49/LConn1
  Ground19/LConn1 -- CC8/LConn1
  C6/RConn1 -- line51/LConn1
  line47/LConn1 -- line50/LConn1
  Current Measurement9/LConn1 -- CC7/RConn1
  Current Measurement7/LConn1 -- CC8/RConn1
  line24/LConn1 -- line42/LConn1 -- line45/RConn1
  line25/LConn1 -- line43/LConn1 -- line46/RConn1
  line26/LConn1 -- line44/LConn1 -- line47/RConn1
  V28/LConn2 -- V29/LConn2 -- Ground32/LConn1 -- V27/LConn2
  line76/RConn1 -- line82/RConn1 -- line83/RConn1
  C8/LConn1 -- V27/LConn1 -- CM14/RConn1 -- Current Measurement12/RConn1 -- line88/LConn1 -- line85/LConn1
  c4/LConn1 -- V29/LConn1 -- CM15/RConn1 -- Current Measurement10/RConn1 -- line89/LConn1 -- line86/LConn1
  line84/LConn1 -- line87/LConn1 -- Current Measurement11/RConn1 -- CM13/RConn1 -- V28/LConn1 -- C7/LConn1
  line85/RConn1 -- line86/RConn1 -- Ground36/LConn1 -- line84/RConn1 -- line87/RConn1 -- line89/RConn1 -- line88/RConn1
  line74/RConn1 -- V26/LConn1 -- CM13/LConn1
  line73/RConn1 -- V30/LConn1 -- CM14/LConn1
  line75/RConn1 -- CM15/LConn1 -- V25/LConn1
  V26/LConn2 -- Ground29/LConn1 -- V30/LConn2
  line62/LConn1 -- line75/LConn1
  Current Measurement12/LConn1 -- CC10/RConn1
  c4/RConn1 -- line83/LConn1
  Ground34/LConn1 -- CC10/LConn1
  Current Measurement10/LConn1 -- CC11/RConn1
  C8/RConn1 -- line76/LConn1
  Ground28/LConn1 -- V25/LConn2
  CC12/LConn1 -- Ground35/LConn1
  C7/RConn1 -- line82/LConn1
  Ground33/LConn1 -- CC11/LConn1
  line60/LConn1 -- line73/LConn1
  Current Measurement11/LConn1 -- CC12/RConn1
  line61/LConn1 -- line74/LConn1

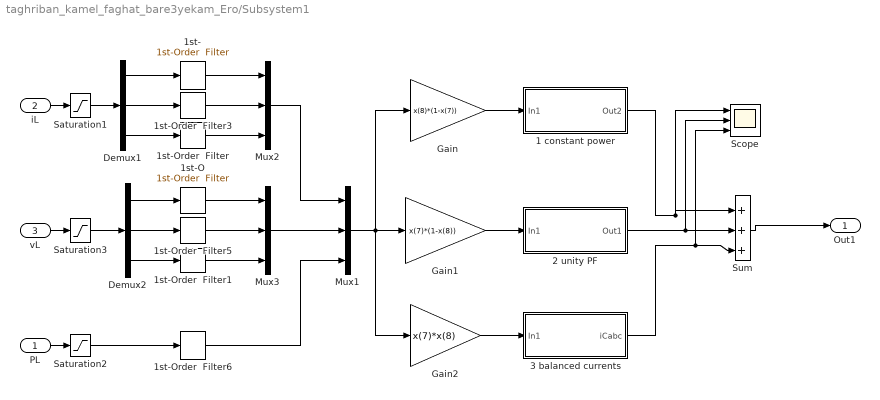
== system taghriban_kamel_faghat_bare3yekam_Ero/Subsystem1 ==
  PL : Inport  OutDataType=fixdt(1, 16)  OutScaling=2^0
  iL : Inport  Port=2  OutDataType=fixdt(1, 16)  OutScaling=2^0
  vL : Inport  Port=3  OutDataType=fixdt(1, 16)  OutScaling=2^0
  1 constant power : Subsystem
  1st- : powerlib_extras/Control  Blocks/1st-Order  Filter  DialogController=POWERSYS.PowerSysDialog  SystemSampleTime=-1  FilterType=Lowpass  Tc=.00051  Initialize=off  Vac_Init=[0.8 -25 60]  Vdc_Init=-0.4  PlotResponse=off  param1=[1 500 1]
  1st-O : powerlib_extras/Control  Blocks/1st-Order  Filter  DialogController=POWERSYS.PowerSysDialog  SystemSampleTime=-1  FilterType=Lowpass  Tc=.00051  Initialize=off  Vac_Init=[0.8 -25 60]  Vdc_Init=-0.4  PlotResponse=off  param1=[1 500 1]
  1st-Order  Filter{,1,3,5..6} (5 alike) : powerlib_extras/Control  Blocks/1st-Order  Filter  DialogController=POWERSYS.PowerSysDialog  SystemSampleTime=-1  FilterType=Lowpass  Tc=.00051  Initialize=off  Vac_Init=[0.8 -25 60]  Vdc_Init=-0.4  PlotResponse=off  param1=[1 500 1]
  2 unity PF : Subsystem
  "3 balanced currents " : Subsystem
  Demux1 : Demux  Outputs=3
  Demux2 : Demux  Outputs=3
  Gain : Gain  Gain=x(8)*(1-x(7))  ParameterDataType=fixdt(1, 16)  ParameterScaling=2^0  OutDataType=fixdt(1, 16)  OutScaling=2^0
  Gain1 : Gain  Gain=x(7)*(1-x(8))  ParameterDataType=fixdt(1, 16)  ParameterScaling=2^0  OutDataType=fixdt(1, 16)  OutScaling=2^0
  Gain2 : Gain  Gain=x(7)*x(8)  ParameterDataType=fixdt(1, 16)  ParameterScaling=2^0  OutDataType=fixdt(1, 16)  OutScaling=2^0
  Mux1 : Mux  Inputs=3
  Mux2 : Mux  Inputs=3
  Mux3 : Mux  Inputs=3
  Saturation1 : Saturate  UpperLimit=100  LowerLimit=-100  OutDataType=sfix(16)  OutScaling=2^0
  Saturation2 : Saturate  UpperLimit=10000  LowerLimit=0  OutDataType=sfix(16)  OutScaling=2^0
  Saturation3 : Saturate  UpperLimit=500  LowerLimit=-500  OutDataType=sfix(16)  OutScaling=2^0
  Scope : Scope  NumInputPorts=3
      settings: YMin=-7.5~-1~-1  YMax=10~1~1  SaveName=ScopeData33
  Sum : Sum  Inputs=|+++  OutDataType=fixdt(1, 16)  OutScaling=2^0
  Out1 : Outport  OutDataType=sfix(16)  OutScaling=2^0
  wires:
  vL/1 -> Saturation3/1
  Demux1/1 -> 1st-/1
  Demux1/2 -> 1st-Order  Filter3/1
  Demux1/3 -> 1st-Order  Filter/1
  Saturation1/1 -> Demux1/1
  1st-Order  Filter1/1 -> Mux3/3
  Demux2/1 -> 1st-O/1
  Demux2/2 -> 1st-Order  Filter5/1
  Demux2/3 -> 1st-Order  Filter1/1
  1st-O/1 -> Mux3/1
  1st-Order  Filter5/1 -> Mux3/2
  Saturation2/1 -> 1st-Order  Filter6/1
  1st-/1 -> Mux2/1
  1st-Order  Filter3/1 -> Mux2/2
  1st-Order  Filter/1 -> Mux2/3
  Saturation3/1 -> Demux2/1
  iL/1 -> Saturation1/1
  PL/1 -> Saturation2/1
  Mux3/1 -> Mux1/2
  Mux2/1 -> Mux1/1
  1st-Order  Filter6/1 -> Mux1/3
  Gain/1 -> 1 constant power/1(In1)
  Mux1/1 -> Gain/1, Gain1/1, Gain2/1
  Gain1/1 -> 2 unity PF/1(In1)
  1 constant power/1(Out2) -> Sum/1, Scope/1
  2 unity PF/1(Out1) -> Sum/2, Scope/2
  Gain2/1 -> "3 balanced currents "/1(In1)
  "3 balanced currents "/1(iCabc) -> Sum/3, Scope/3
  Sum/1 -> Out1/1

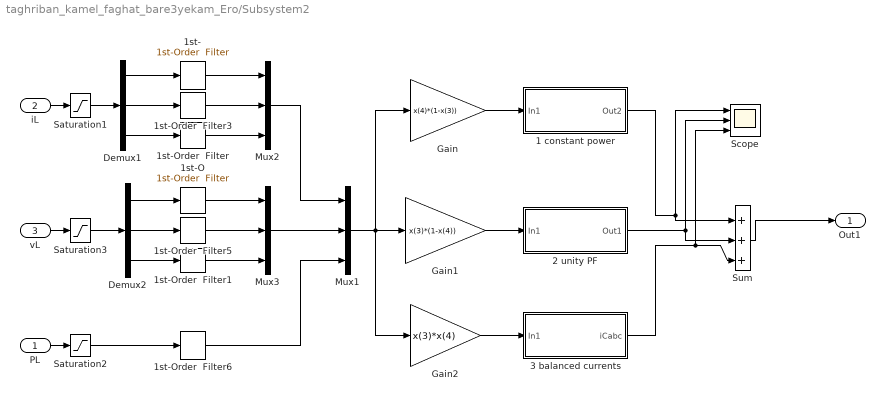
== system taghriban_kamel_faghat_bare3yekam_Ero/Subsystem2 ==
  PL : Inport  OutDataType=fixdt(1, 16)  OutScaling=2^0
  iL : Inport  Port=2  OutDataType=fixdt(1, 16)  OutScaling=2^0
  vL : Inport  Port=3  OutDataType=fixdt(1, 16)  OutScaling=2^0
  1 constant power : Subsystem
  1st- : powerlib_extras/Control  Blocks/1st-Order  Filter  DialogController=POWERSYS.PowerSysDialog  SystemSampleTime=-1  FilterType=Lowpass  Tc=.00051  Initialize=off  Vac_Init=[0.8 -25 60]  Vdc_Init=-0.4  PlotResponse=off  param1=[1 500 1]
  1st-O : powerlib_extras/Control  Blocks/1st-Order  Filter  DialogController=POWERSYS.PowerSysDialog  SystemSampleTime=-1  FilterType=Lowpass  Tc=.00051  Initialize=off  Vac_Init=[0.8 -25 60]  Vdc_Init=-0.4  PlotResponse=off  param1=[1 500 1]
  1st-Order  Filter{,1,3,5..6} (5 alike) : powerlib_extras/Control  Blocks/1st-Order  Filter  DialogController=POWERSYS.PowerSysDialog  SystemSampleTime=-1  FilterType=Lowpass  Tc=.00051  Initialize=off  Vac_Init=[0.8 -25 60]  Vdc_Init=-0.4  PlotResponse=off  param1=[1 500 1]
  2 unity PF : Subsystem
  "3 balanced currents " : Subsystem
  Demux1 : Demux  Outputs=3
  Demux2 : Demux  Outputs=3
  Gain : Gain  Gain=x(4)*(1-x(3))  ParameterDataType=fixdt(1, 16)  ParameterScaling=2^0  OutDataType=fixdt(1, 16)  OutScaling=2^0
  Gain1 : Gain  Gain=x(3)*(1-x(4))  ParameterDataType=fixdt(1, 16)  ParameterScaling=2^0  OutDataType=fixdt(1, 16)  OutScaling=2^0
  Gain2 : Gain  Gain=x(3)*x(4)  ParameterDataType=fixdt(1, 16)  ParameterScaling=2^0  OutDataType=fixdt(1, 16)  OutScaling=2^0
  Mux1 : Mux  Inputs=3
  Mux2 : Mux  Inputs=3
  Mux3 : Mux  Inputs=3
  Saturation1 : Saturate  UpperLimit=100  LowerLimit=-100  OutDataType=sfix(16)  OutScaling=2^0
  Saturation2 : Saturate  UpperLimit=10000  LowerLimit=0  OutDataType=sfix(16)  OutScaling=2^0
  Saturation3 : Saturate  UpperLimit=500  LowerLimit=-500  OutDataType=sfix(16)  OutScaling=2^0
  Scope : Scope  NumInputPorts=3
      settings: YMin=-7.5~-1~-1  YMax=10~1~1  SaveName=ScopeData33
  Sum : Sum  Inputs=|+++  OutDataType=fixdt(1, 16)  OutScaling=2^0
  Out1 : Outport  OutDataType=sfix(16)  OutScaling=2^0
  wires:
  vL/1 -> Saturation3/1
  Demux1/1 -> 1st-/1
  Demux1/2 -> 1st-Order  Filter3/1
  Demux1/3 -> 1st-Order  Filter/1
  Saturation1/1 -> Demux1/1
  1st-Order  Filter1/1 -> Mux3/3
  Demux2/1 -> 1st-O/1
  Demux2/2 -> 1st-Order  Filter5/1
  Demux2/3 -> 1st-Order  Filter1/1
  1st-O/1 -> Mux3/1
  1st-Order  Filter5/1 -> Mux3/2
  Saturation2/1 -> 1st-Order  Filter6/1
  1st-/1 -> Mux2/1
  1st-Order  Filter3/1 -> Mux2/2
  1st-Order  Filter/1 -> Mux2/3
  Saturation3/1 -> Demux2/1
  iL/1 -> Saturation1/1
  PL/1 -> Saturation2/1
  Mux3/1 -> Mux1/2
  Mux2/1 -> Mux1/1
  1st-Order  Filter6/1 -> Mux1/3
  Gain/1 -> 1 constant power/1(In1)
  Mux1/1 -> Gain/1, Gain1/1, Gain2/1
  Gain1/1 -> 2 unity PF/1(In1)
  1 constant power/1(Out2) -> Sum/1, Scope/1
  2 unity PF/1(Out1) -> Sum/2, Scope/2
  Gain2/1 -> "3 balanced currents "/1(In1)
  "3 balanced currents "/1(iCabc) -> Sum/3, Scope/3
  Sum/1 -> Out1/1

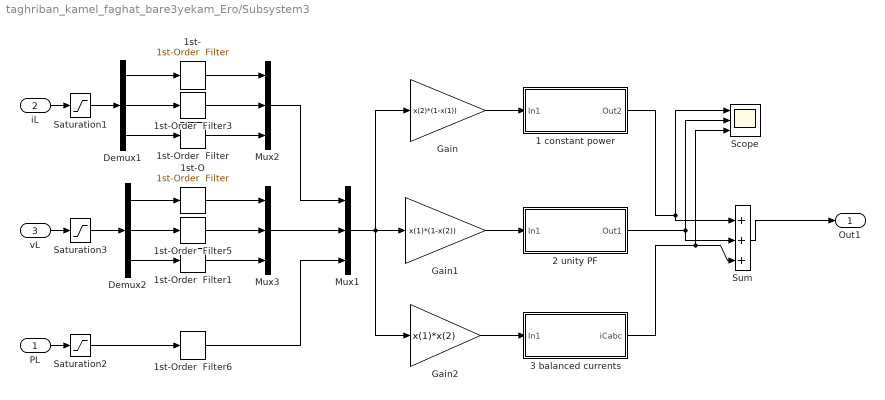
== system taghriban_kamel_faghat_bare3yekam_Ero/Subsystem3 ==
  PL : Inport  OutDataType=fixdt(1, 16)  OutScaling=2^0
  iL : Inport  Port=2  OutDataType=fixdt(1, 16)  OutScaling=2^0
  vL : Inport  Port=3  OutDataType=fixdt(1, 16)  OutScaling=2^0
  1 constant power : Subsystem
  1st- : powerlib_extras/Control  Blocks/1st-Order  Filter  DialogController=POWERSYS.PowerSysDialog  SystemSampleTime=-1  FilterType=Lowpass  Tc=.00051  Initialize=off  Vac_Init=[0.8 -25 60]  Vdc_Init=-0.4  PlotResponse=off  param1=[1 500 1]
  1st-O : powerlib_extras/Control  Blocks/1st-Order  Filter  DialogController=POWERSYS.PowerSysDialog  SystemSampleTime=-1  FilterType=Lowpass  Tc=.00051  Initialize=off  Vac_Init=[0.8 -25 60]  Vdc_Init=-0.4  PlotResponse=off  param1=[1 500 1]
  1st-Order  Filter{,1,3,5..6} (5 alike) : powerlib_extras/Control  Blocks/1st-Order  Filter  DialogController=POWERSYS.PowerSysDialog  SystemSampleTime=-1  FilterType=Lowpass  Tc=.00051  Initialize=off  Vac_Init=[0.8 -25 60]  Vdc_Init=-0.4  PlotResponse=off  param1=[1 500 1]
  2 unity PF : Subsystem
  "3 balanced currents " : Subsystem
  Demux1 : Demux  Outputs=3
  Demux2 : Demux  Outputs=3
  Gain : Gain  Gain=x(2)*(1-x(1))  ParameterDataType=fixdt(1, 16)  ParameterScaling=2^0  OutDataType=fixdt(1, 16)  OutScaling=2^0
  Gain1 : Gain  Gain=x(1)*(1-x(2))  ParameterDataType=fixdt(1, 16)  ParameterScaling=2^0  OutDataType=fixdt(1, 16)  OutScaling=2^0
  Gain2 : Gain  Gain=x(1)*x(2)  ParameterDataType=fixdt(1, 16)  ParameterScaling=2^0  OutDataType=fixdt(1, 16)  OutScaling=2^0
  Mux1 : Mux  Inputs=3
  Mux2 : Mux  Inputs=3
  Mux3 : Mux  Inputs=3
  Saturation1 : Saturate  UpperLimit=100  LowerLimit=-100  OutDataType=sfix(16)  OutScaling=2^0
  Saturation2 : Saturate  UpperLimit=10000  LowerLimit=0  OutDataType=sfix(16)  OutScaling=2^0
  Saturation3 : Saturate  UpperLimit=500  LowerLimit=-500  OutDataType=sfix(16)  OutScaling=2^0
  Scope : Scope  NumInputPorts=3
      settings: YMin=-7.5~-1~-1  YMax=10~1~1  SaveName=ScopeData33
  Sum : Sum  Inputs=|+++  OutDataType=fixdt(1, 16)  OutScaling=2^0
  Out1 : Outport  OutDataType=sfix(16)  OutScaling=2^0
  wires:
  vL/1 -> Saturation3/1
  Demux1/1 -> 1st-/1
  Demux1/2 -> 1st-Order  Filter3/1
  Demux1/3 -> 1st-Order  Filter/1
  Saturation1/1 -> Demux1/1
  1st-Order  Filter1/1 -> Mux3/3
  Demux2/1 -> 1st-O/1
  Demux2/2 -> 1st-Order  Filter5/1
  Demux2/3 -> 1st-Order  Filter1/1
  1st-O/1 -> Mux3/1
  1st-Order  Filter5/1 -> Mux3/2
  Saturation2/1 -> 1st-Order  Filter6/1
  1st-/1 -> Mux2/1
  1st-Order  Filter3/1 -> Mux2/2
  1st-Order  Filter/1 -> Mux2/3
  Saturation3/1 -> Demux2/1
  iL/1 -> Saturation1/1
  PL/1 -> Saturation2/1
  Mux3/1 -> Mux1/2
  Mux2/1 -> Mux1/1
  1st-Order  Filter6/1 -> Mux1/3
  Gain/1 -> 1 constant power/1(In1)
  Mux1/1 -> Gain/1, Gain1/1, Gain2/1
  Gain1/1 -> 2 unity PF/1(In1)
  1 constant power/1(Out2) -> Sum/1, Scope/1
  2 unity PF/1(Out1) -> Sum/2, Scope/2
  Gain2/1 -> "3 balanced currents "/1(In1)
  "3 balanced currents "/1(iCabc) -> Sum/3, Scope/3
  Sum/1 -> Out1/1

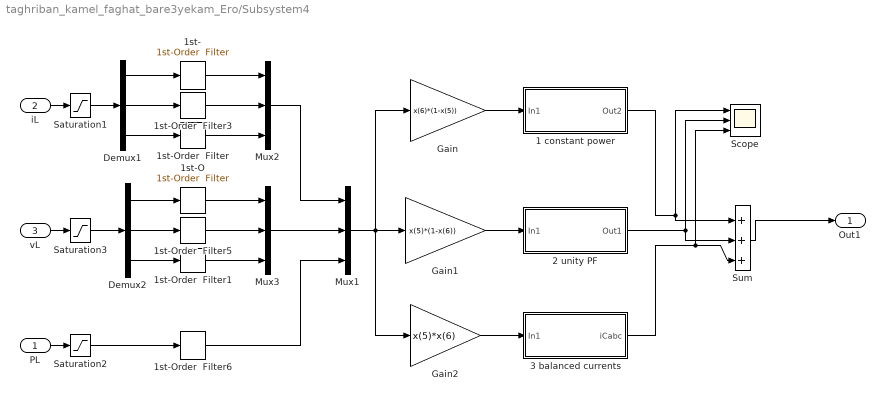
== system taghriban_kamel_faghat_bare3yekam_Ero/Subsystem4 ==
  PL : Inport  OutDataType=fixdt(1, 16)  OutScaling=2^0
  iL : Inport  Port=2  OutDataType=fixdt(1, 16)  OutScaling=2^0
  vL : Inport  Port=3  OutDataType=fixdt(1, 16)  OutScaling=2^0
  1 constant power : Subsystem
  1st- : powerlib_extras/Control  Blocks/1st-Order  Filter  DialogController=POWERSYS.PowerSysDialog  SystemSampleTime=-1  FilterType=Lowpass  Tc=.00051  Initialize=off  Vac_Init=[0.8 -25 60]  Vdc_Init=-0.4  PlotResponse=off  param1=[1 500 1]
  1st-O : powerlib_extras/Control  Blocks/1st-Order  Filter  DialogController=POWERSYS.PowerSysDialog  SystemSampleTime=-1  FilterType=Lowpass  Tc=.00051  Initialize=off  Vac_Init=[0.8 -25 60]  Vdc_Init=-0.4  PlotResponse=off  param1=[1 500 1]
  1st-Order  Filter{,1,3,5..6} (5 alike) : powerlib_extras/Control  Blocks/1st-Order  Filter  DialogController=POWERSYS.PowerSysDialog  SystemSampleTime=-1  FilterType=Lowpass  Tc=.00051  Initialize=off  Vac_Init=[0.8 -25 60]  Vdc_Init=-0.4  PlotResponse=off  param1=[1 500 1]
  2 unity PF : Subsystem
  "3 balanced currents " : Subsystem
  Demux1 : Demux  Outputs=3
  Demux2 : Demux  Outputs=3
  Gain : Gain  Gain=x(6)*(1-x(5))  ParameterDataType=fixdt(1, 16)  ParameterScaling=2^0  OutDataType=fixdt(1, 16)  OutScaling=2^0
  Gain1 : Gain  Gain=x(5)*(1-x(6))  ParameterDataType=fixdt(1, 16)  ParameterScaling=2^0  OutDataType=fixdt(1, 16)  OutScaling=2^0
  Gain2 : Gain  Gain=x(5)*x(6)  ParameterDataType=fixdt(1, 16)  ParameterScaling=2^0  OutDataType=fixdt(1, 16)  OutScaling=2^0
  Mux1 : Mux  Inputs=3
  Mux2 : Mux  Inputs=3
  Mux3 : Mux  Inputs=3
  Saturation1 : Saturate  UpperLimit=100  LowerLimit=-100  OutDataType=sfix(16)  OutScaling=2^0
  Saturation2 : Saturate  UpperLimit=10000  LowerLimit=0  OutDataType=sfix(16)  OutScaling=2^0
  Saturation3 : Saturate  UpperLimit=500  LowerLimit=-500  OutDataType=sfix(16)  OutScaling=2^0
  Scope : Scope  NumInputPorts=3
      settings: YMin=-7.5~-1~-1  YMax=10~1~1  SaveName=ScopeData33
  Sum : Sum  Inputs=|+++  OutDataType=fixdt(1, 16)  OutScaling=2^0
  Out1 : Outport  OutDataType=sfix(16)  OutScaling=2^0
  wires:
  vL/1 -> Saturation3/1
  Demux1/1 -> 1st-/1
  Demux1/2 -> 1st-Order  Filter3/1
  Demux1/3 -> 1st-Order  Filter/1
  Saturation1/1 -> Demux1/1
  1st-Order  Filter1/1 -> Mux3/3
  Demux2/1 -> 1st-O/1
  Demux2/2 -> 1st-Order  Filter5/1
  Demux2/3 -> 1st-Order  Filter1/1
  1st-O/1 -> Mux3/1
  1st-Order  Filter5/1 -> Mux3/2
  Saturation2/1 -> 1st-Order  Filter6/1
  1st-/1 -> Mux2/1
  1st-Order  Filter3/1 -> Mux2/2
  1st-Order  Filter/1 -> Mux2/3
  Saturation3/1 -> Demux2/1
  iL/1 -> Saturation1/1
  PL/1 -> Saturation2/1
  Mux3/1 -> Mux1/2
  Mux2/1 -> Mux1/1
  1st-Order  Filter6/1 -> Mux1/3
  Gain/1 -> 1 constant power/1(In1)
  Mux1/1 -> Gain/1, Gain1/1, Gain2/1
  Gain1/1 -> 2 unity PF/1(In1)
  1 constant power/1(Out2) -> Sum/1, Scope/1
  2 unity PF/1(Out1) -> Sum/2, Scope/2
  Gain2/1 -> "3 balanced currents "/1(In1)
  "3 balanced currents "/1(iCabc) -> Sum/3, Scope/3
  Sum/1 -> Out1/1
